simulink model "Impedance_model"  (R2021a)
settings: Solver=FixedStepDiscrete  StartTime=0.0  StopTime=Tfinal  FixedStep=SampleTime  RelTol=1e-3
InitFcn:
  | param
values from neighbouring files (symbols this model uses):
  Cp = 28.5e-9    (= 2.85e-08)    [WPT_resistance_multiple.m]    (also in analytical_model.m; param.m)
  Cs = 115e-9    (= 1.15e-07)    [WPT_resistance_multiple.m]    (also in analytical_model.m; param.m)
  Lmotor = 1e-3    (= 0.001)    [WPT_resistance_multiple.m]    (also in analytical_model.m; param.m)
  Lp = 205e-6    (= 0.000205)    [WPT_resistance_multiple.m]    (also in analytical_model.m; param.m)
  Ls = 51e-6    (= 5.1e-05)    [WPT_resistance_multiple.m]    (also in analytical_model.m; param.m)
  M = 41e-6    (= 4.1e-05)    [WPT_resistance_multiple.m]    (also in analytical_model.m; param.m)
  RL = RLk(i)    [WPT_resistance_multiple.m]    (also in analytical_model.m = 8.44; param.m = 8.44)
  Rmotor = 2    [WPT_resistance_multiple.m]    (also in analytical_model.m; param.m)
  SampleTime = (1/fsw)/360    (= 3.08641975309e-08)    [param.m]
libraries: spsSeriesRLCBranchLib x18, spsImpedanceMeasurementLib x2, spsControlledVoltageSourceLib x1, spsCurrentMeasurementLib x1, spsVoltageMeasurementLib x1, spspowerguiLib x1
settings Model: Creator=enes_  LastModifiedBy=enes_
settings SolverCC: AlgebraicLoopSolver=TrustRegion
settings DataIOCC: ReturnWorkspaceOutputs=off
settings DebuggingCC: UnconnectedLineMsg=none  SFMachineParentedDataDiag=warning  ArithmeticOperatorsInVariantConditions=warning
settings SFSimCC: SimUseLocalCustomCode=off  CustomCodeUndefinedFunction=UseInterfaceOnly
settings RTWCC: RTWUseLocalCustomCode=off

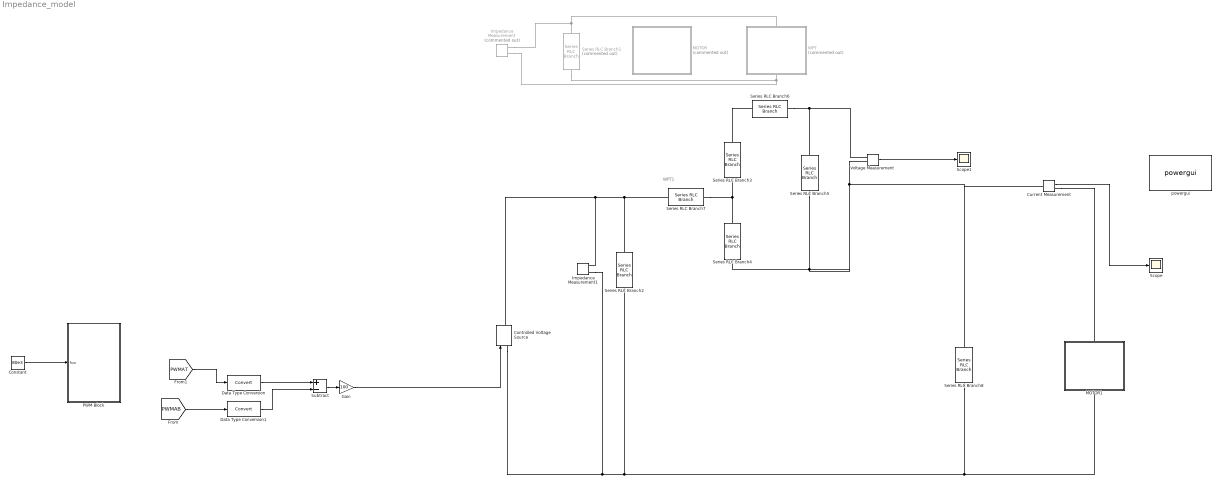
== system Impedance_model ==
  note: WPT1
  Constant : Constant  Value=80e3
  Controlled Voltage Source : spsControlledVoltageSourceLib/Controlled Voltage Source  Initialize=on  Source_Type=AC  Amplitude=0  Phase=0  Frequency=0  Measurements=None
  Current Measurement : spsCurrentMeasurementLib/Current Measurement  PhasorSimulation=off  OutputType=Complex  PSBequivalent=0
  Data Type Conversion : DataTypeConversion
  Data Type Conversion1 : DataTypeConversion
  Gain : Gain  Gain=100
  Impedance Measurement : spsImpedanceMeasurementLib/Impedance Measurement  Commented=on  LConnTagsString=+|-  Factor=1
      settings: SourceProductBaseCode=PS
  Impedance Measurement1 : spsImpedanceMeasurementLib/Impedance Measurement  LConnTagsString=+|-  Factor=1
      settings: SourceProductBaseCode=PS
  MOTOR : Subsystem  Commented=on
  MOTOR1 : Subsystem
  PWM Block : Subsystem
  Scope : Scope
  Scope1 : Scope
  Series RLC Branch1 : spsSeriesRLCBranchLib/Series RLC Branch  Commented=on  LConnTagsString=__new0  RConnTagsString=__new0  BranchType=R  Resistance=1e6  Inductance=Lp-M  SetiL0=off  InitialCurrent=0  Capacitance=Cp  Setx0=off  InitialVoltage=0  Measurements=None
  Series RLC Branch2 : spsSeriesRLCBranchLib/Series RLC Branch  LConnTagsString=__new0  RConnTagsString=__new0  BranchType=R  Resistance=1e6  Inductance=Lp-M  SetiL0=off  InitialCurrent=0  Capacitance=Cp  Setx0=off  InitialVoltage=0  Measurements=None
  Series RLC Branch3 : spsSeriesRLCBranchLib/Series RLC Branch  LConnTagsString=__new0  RConnTagsString=__new0  BranchType=L  Resistance=1  Inductance=Ls-M  SetiL0=off  InitialCurrent=0  Capacitance=Cp  Setx0=off  InitialVoltage=0  Measurements=None
  Series RLC Branch4 : spsSeriesRLCBranchLib/Series RLC Branch  LConnTagsString=__new0  RConnTagsString=__new0  BranchType=L  Resistance=1  Inductance=Lp-M  SetiL0=off  InitialCurrent=0  Capacitance=Cp  Setx0=off  InitialVoltage=0  Measurements=None
  Series RLC Branch5 : spsSeriesRLCBranchLib/Series RLC Branch  LConnTagsString=__new0  RConnTagsString=__new0  BranchType=R  Resistance=RL  Inductance=Ls-M  SetiL0=off  InitialCurrent=0  Capacitance=Cp  Setx0=off  InitialVoltage=0  Measurements=None
  Series RLC Branch6 : spsSeriesRLCBranchLib/Series RLC Branch  LConnTagsString=__new0  RConnTagsString=__new0  BranchType=C  Resistance=1  Inductance=1e-3  SetiL0=off  InitialCurrent=0  Capacitance=Cs  Setx0=off  InitialVoltage=0  Measurements=None
  Series RLC Branch7 : spsSeriesRLCBranchLib/Series RLC Branch  LConnTagsString=__new0  RConnTagsString=__new0  BranchType=L  Resistance=1  Inductance=Lp-M  SetiL0=off  InitialCurrent=0  Capacitance=Cp  Setx0=off  InitialVoltage=0  Measurements=None
  Series RLC Branch8 : spsSeriesRLCBranchLib/Series RLC Branch  LConnTagsString=__new0  RConnTagsString=__new0  BranchType=C  Resistance=1  Inductance=1e-3  SetiL0=off  InitialCurrent=0  Capacitance=100e-6  Setx0=off  InitialVoltage=0  Measurements=None
  Subtract : Sum  Inputs=+-
  Voltage Measurement : spsVoltageMeasurementLib/Voltage Measurement  PhasorSimulation=off  OutputType=Complex  PSBequivalent=0
  WPT : Subsystem  Commented=on
  powergui : spspowerguiLib/powergui  Priority=1  SimulationMode=Discrete  SampleTime=SampleTime  frequency=60  Iterations=50  frequencyindice=60  Pbase=100e6  ErrMax=1e-4  UnitsV=kV  UnitsW=MW  buscounter=0  FunctionMessages=off  echomessages=off  EnableUseOfTLC=off  CurrentSourceSwitches=off  DisableSnubberDevices=off  DisableRonSwitches=off  DisableVfSwitches=off  DisplayEquations=off  AutomaticDiscreteSolvers=off  SolverType=Tustin/Backward Euler (TBE)  Interpol=off  ExternalGateDelay=off  methode=off  Ts=100  x0status=blocks  SPID=on  SwTol=0  HookPort=off  NonlinearTolerance=1e-4  nMaxIteration=100  ContinueOnMaxIteration=off  RestoreLinks=warning  ResistiveCurrentMeasurement=off  Frange=[0:1e3:1e6]  Ylog=on  Xlog=on  ShowGrid=off  save=off  variable=ZData  structure=inputVoltage  ZoomFFT=off  StartTime=0.0  cycles=100  DisplayStyle=1  fundamental=80000  FreqAxis=off  MaxFrequency=240e3  frequencyindicesteady=1  RmsSteady=1  display=off
  wires:
  Constant/1 -> PWM Block/1(fsw)
  [PWMAT] -> Data Type Conversion/1
  [PWMAB] -> Data Type Conversion1/1
  Subtract/1 -> Gain/1
  Gain/1 -> Controlled Voltage Source/1
  Current Measurement/1 -> Scope/1
  Voltage Measurement/1 -> Scope1/1
  Data Type Conversion/1 -> Subtract/1
  Data Type Conversion1/1 -> Subtract/2
  connections:
  WPT/LConn1 -- Series RLC Branch1/LConn1 -- Impedance Measurement/LConn1
  WPT/RConn1 -- Series RLC Branch1/RConn1 -- Impedance Measurement/LConn2
  Impedance Measurement1/LConn2 -- Series RLC Branch2/RConn1 -- Series RLC Branch8/LConn1 -- MOTOR1/RConn1 -- Controlled Voltage Source/LConn1
  Series RLC Branch6/LConn1 -- Voltage Measurement/LConn1 -- Series RLC Branch5/LConn1
  Series RLC Branch4/LConn1 -- Series RLC Branch7/RConn1 -- Series RLC Branch3/LConn1
  Series RLC Branch3/RConn1 -- Series RLC Branch6/RConn1
  Impedance Measurement1/LConn1 -- Series RLC Branch7/LConn1 -- Series RLC Branch2/LConn1 -- Controlled Voltage Source/RConn1
  Series RLC Branch5/RConn1 -- Series RLC Branch8/RConn1 -- Current Measurement/LConn1 -- Voltage Measurement/LConn2 -- Series RLC Branch4/RConn1
  Current Measurement/RConn1 -- MOTOR1/LConn1

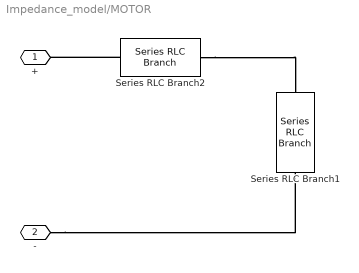
== system Impedance_model/MOTOR ==
  Series RLC Branch1 : spsSeriesRLCBranchLib/Series RLC Branch  LConnTagsString=__new0  RConnTagsString=__new0  BranchType=R  Resistance=Rmotor  Inductance=Lp-M  SetiL0=off  InitialCurrent=0  Capacitance=Cp  Setx0=off  InitialVoltage=0  Measurements=None
  Series RLC Branch2 : spsSeriesRLCBranchLib/Series RLC Branch  LConnTagsString=__new0  RConnTagsString=__new0  BranchType=L  Resistance=1  Inductance=Lmotor  SetiL0=off  InitialCurrent=0  Capacitance=Cp  Setx0=off  InitialVoltage=0  Measurements=None
  + : PMIOPort  Side=Left
  - : PMIOPort  Port=2  Side=Right
  connections:
  -/RConn1 -- Series RLC Branch1/RConn1
  Series RLC Branch2/RConn1 -- Series RLC Branch1/LConn1
  Series RLC Branch2/LConn1 -- +/RConn1

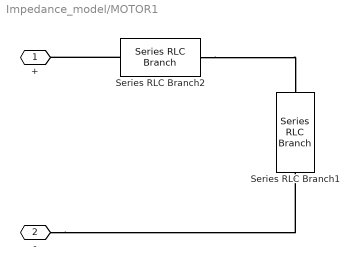
== system Impedance_model/MOTOR1 ==
  Series RLC Branch1 : spsSeriesRLCBranchLib/Series RLC Branch  LConnTagsString=__new0  RConnTagsString=__new0  BranchType=R  Resistance=Rmotor  Inductance=Lp-M  SetiL0=off  InitialCurrent=0  Capacitance=Cp  Setx0=off  InitialVoltage=0  Measurements=None
  Series RLC Branch2 : spsSeriesRLCBranchLib/Series RLC Branch  LConnTagsString=__new0  RConnTagsString=__new0  BranchType=L  Resistance=1  Inductance=Lmotor  SetiL0=off  InitialCurrent=0  Capacitance=Cp  Setx0=off  InitialVoltage=0  Measurements=None
  + : PMIOPort  Side=Left
  - : PMIOPort  Port=2  Side=Right
  connections:
  -/RConn1 -- Series RLC Branch1/RConn1
  Series RLC Branch2/RConn1 -- Series RLC Branch1/LConn1
  Series RLC Branch2/LConn1 -- +/RConn1

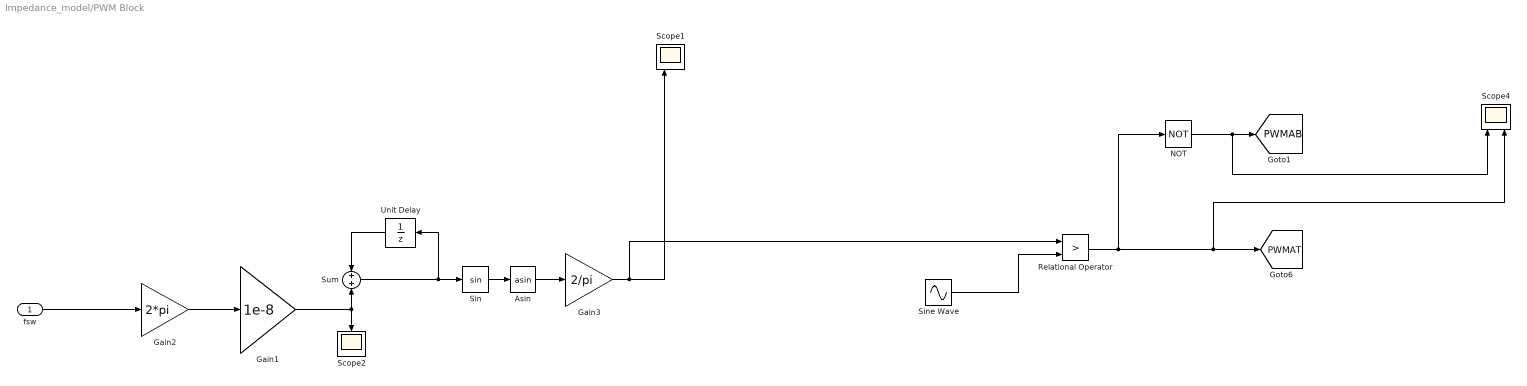
== system Impedance_model/PWM Block ==
  fsw : Inport
  Asin : Trigonometry  Operator=asin
  Gain1 : Gain  Gain=1e-8
  Gain2 : Gain  Gain=2*pi
  Gain3 : Gain  Gain=2/pi
  NOT : Logic  Operator=NOT  IconShape=distinctive  AllPortsSameDT=off  OutDataTypeStr=boolean
  Relational Operator : RelationalOperator  Operator=>  OutDataTypeStr=boolean  RndMeth=Simplest
  Scope1 : Scope  NumInputPorts=2
  Scope2 : Scope
  Scope4 : Scope  NumInputPorts=3
  Sin : Trigonometry
  Sine Wave : Sin  Amplitude=0.8  Frequency=50*2*pi  SampleTime=0
  Sum : Sum
  Unit Delay : UnitDelay  SampleTime=-1  HasFrameUpgradeWarning=on
  tag scope: PWMAB=global, PWMAT=global
  wires:
  NOT/1 -> Scope4/1, [PWMAB]
  Relational Operator/1 -> NOT/1, Scope4/3, [PWMAT]
  Sin/1 -> Asin/1
  Asin/1 -> Gain3/1
  Sum/1 -> Sin/1, Unit Delay/1
  Unit Delay/1 -> Sum/1
  Gain2/1 -> Gain1/1
  Gain1/1 -> Sum/2, Scope2/1
  fsw/1 -> Gain2/1
  Gain3/1 -> Relational Operator/1, Scope1/1
  Sine Wave/1 -> Relational Operator/2

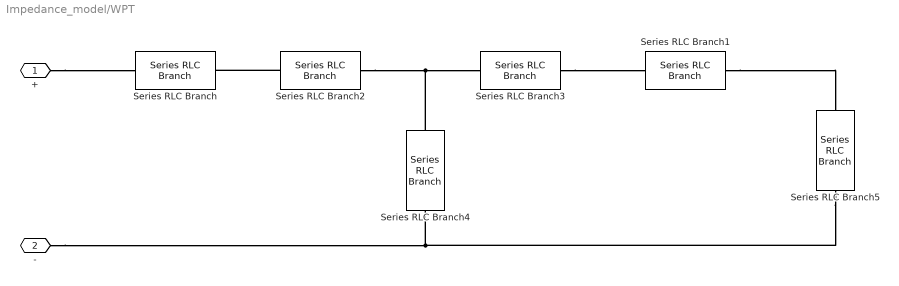
== system Impedance_model/WPT ==
  Series RLC Branch : spsSeriesRLCBranchLib/Series RLC Branch  LConnTagsString=__new0  RConnTagsString=__new0  BranchType=C  Resistance=1  Inductance=1e-3  SetiL0=off  InitialCurrent=0  Capacitance=Cp  Setx0=off  InitialVoltage=0  Measurements=None
  Series RLC Branch1 : spsSeriesRLCBranchLib/Series RLC Branch  LConnTagsString=__new0  RConnTagsString=__new0  BranchType=C  Resistance=1  Inductance=1e-3  SetiL0=off  InitialCurrent=0  Capacitance=Cs  Setx0=off  InitialVoltage=0  Measurements=None
  Series RLC Branch2 : spsSeriesRLCBranchLib/Series RLC Branch  LConnTagsString=__new0  RConnTagsString=__new0  BranchType=L  Resistance=1  Inductance=Lp-M  SetiL0=off  InitialCurrent=0  Capacitance=Cp  Setx0=off  InitialVoltage=0  Measurements=None
  Series RLC Branch3 : spsSeriesRLCBranchLib/Series RLC Branch  LConnTagsString=__new0  RConnTagsString=__new0  BranchType=L  Resistance=1  Inductance=Ls-M  SetiL0=off  InitialCurrent=0  Capacitance=Cp  Setx0=off  InitialVoltage=0  Measurements=None
  Series RLC Branch4 : spsSeriesRLCBranchLib/Series RLC Branch  LConnTagsString=__new0  RConnTagsString=__new0  BranchType=L  Resistance=1  Inductance=Lp-M  SetiL0=off  InitialCurrent=0  Capacitance=Cp  Setx0=off  InitialVoltage=0  Measurements=None
  Series RLC Branch5 : spsSeriesRLCBranchLib/Series RLC Branch  LConnTagsString=__new0  RConnTagsString=__new0  BranchType=R  Resistance=RL  Inductance=Ls-M  SetiL0=off  InitialCurrent=0  Capacitance=Cp  Setx0=off  InitialVoltage=0  Measurements=None
  + : PMIOPort  Side=Left
  - : PMIOPort  Port=2  Side=Right
  connections:
  -/RConn1 -- Series RLC Branch5/RConn1 -- Series RLC Branch4/RConn1
  Series RLC Branch2/LConn1 -- Series RLC Branch/RConn1
  Series RLC Branch3/RConn1 -- Series RLC Branch1/RConn1
  Series RLC Branch4/LConn1 -- Series RLC Branch2/RConn1 -- Series RLC Branch3/LConn1
  Series RLC Branch1/LConn1 -- Series RLC Branch5/LConn1
  +/RConn1 -- Series RLC Branch/LConn1
